simulink model "Maths_Eqn"  (R2022b)
settings: Solver=VariableStepAuto  StartTime=0.0  StopTime=10.0  RelTol=1e-3
values from neighbouring files (symbols this model uses):
  A = 3    [Project_2.m]
  F = 2    [Project_2.m]
  Ti = 0.5    [Project_2.m]
settings Model: Creator=Ayush Pharande  LastModifiedBy=Ayush Pharande

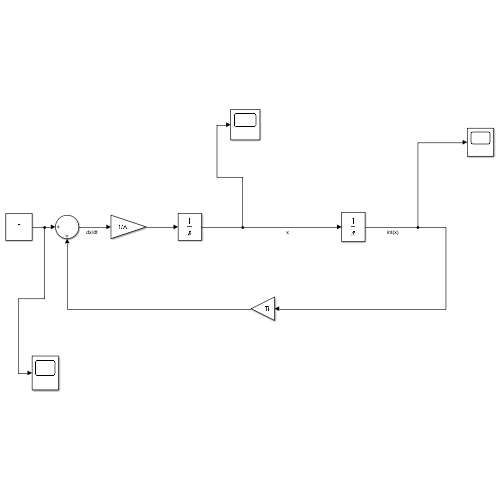
[thumbnail: Simulink's stored preview of the top-level diagram]
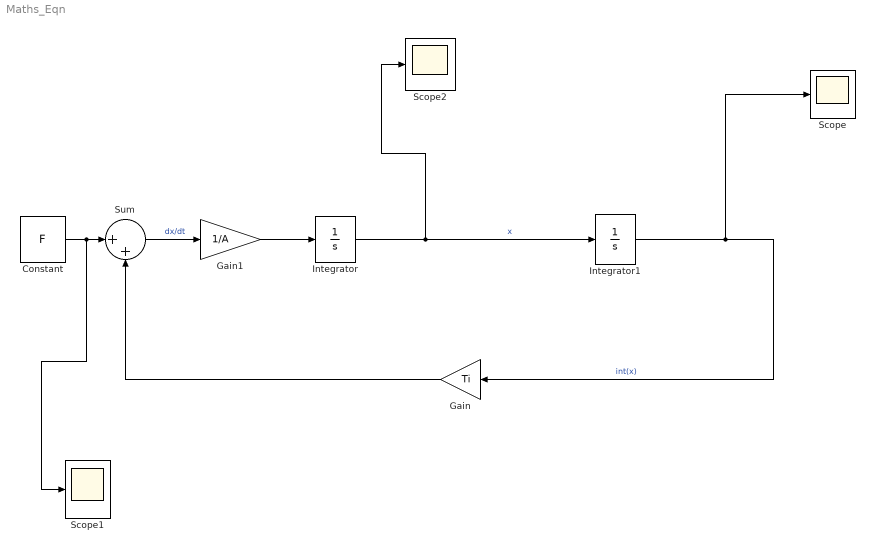
== system Maths_Eqn ==
  Constant : Constant  Value=F
  Gain : Gain  Gain=Ti
  Gain1 : Gain  Gain=1/A
  Integrator : Integrator
  Integrator1 : Integrator
  Scope : Scope
  Scope1 : Scope
  Scope2 : Scope
  Sum : Sum  Inputs=|++
  wires:
  Integrator/1 -> Scope2/1, Integrator1/1  "x"
  Sum/1 -> Gain1/1  "dx/dt"
  Integrator1/1 -> Scope/1, Gain/1  "int(x)"
  Gain1/1 -> Integrator/1
  Constant/1 -> Scope1/1, Sum/1
  Gain/1 -> Sum/2
